simulink model "Test Trajectory"  (R2020a)
settings: Solver=VariableStepAuto  StartTime=0.0  StopTime=10.0  RelTol=1e-3
libraries: simulink x2
settings Model: Creator=ashut  LastModifiedBy=ashut

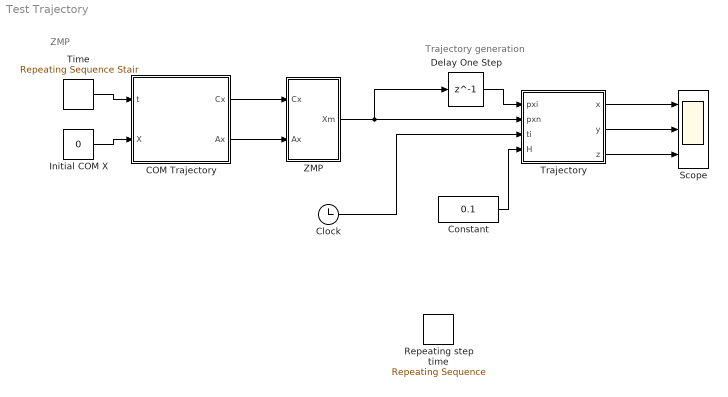
== system Test Trajectory ==
  note: Trajectory generation
  note: ZMP
  COM Trajectory : MATLAB Function  TreatAsAtomicUnit=on
  Clock : Clock
  Constant : Constant  Value=0.1
  Delay One Step : Delay  DelayLength=1
  Initial COM X : Constant  Value=0
  Repeating step time : simulink/Sources/Repeating Sequence  rep_seq_t=[0 0.5]  rep_seq_y=[0 0.5]
  Scope : Scope  NumInputPorts=3
  Time : simulink/Sources/Repeating Sequence Stair  OutValues=[0:1:10].'  tsamp=1  OutMin=[]  OutMax=[]  OutDataTypeStr=double  OutputDataTypeScalingMode=double  OutDataType=fixdt(0,8)  ConRadixGroup=Best Precision: Vector-wise  OutScaling=2^-12
  Trajectory : MATLAB Function  TreatAsAtomicUnit=on
  ZMP : MATLAB Function  TreatAsAtomicUnit=on
  wires:
  COM Trajectory/1(Cx) -> ZMP/1(Cx)
  Constant/1 -> Trajectory/4(H)
  ZMP/1(Xm) -> Delay One Step/1, Trajectory/2(pxn)
  Time/1 -> COM Trajectory/1(t)
  Initial COM X/1 -> COM Trajectory/2(X)
  Delay One Step/1 -> Trajectory/1(pxi)
  COM Trajectory/2(Ax) -> ZMP/2(Ax)
  Trajectory/1(x) -> Scope/1
  Trajectory/2(y) -> Scope/2
  Trajectory/3(z) -> Scope/3
  Clock/1 -> Trajectory/3(ti)

== matlab function Test Trajectory/Trajectory ==
  data: x output; y output; pxi input; z output; pxn input; ti input; H input
function[x,y,z] = Trajectory(pxi,pxn,ti,H)
% pxi is cuttrent x position of endpoint
% pxn is final x position of enpoint
% ti is the real time
% H is the height of the step

% These all are in world frame
step_time = 0.5;
x = pxi + sin((pi/2*step_time)*ti)*abs(pxn-pxi);
y = 0;
z = sin((pi/step_time)*ti)*(H);

== matlab function Test Trajectory/ZMP ==
  data: Cx input; Ax input; Xm output
function Xm  = ZMP(Cx,Ax)

% g and h defined in Parameters.m
% h here is COM height(z-cordinate) from world/path
h = 0.25;
g = 9.8066;
Xm = Cx - (h/g)*(Ax);

== matlab function Test Trajectory/COM Trajectory ==
  data: t input; Cx output; X input; Ax output
function[Cx,Ax] = COM_Trajectory(t,X)
% Here t is sample time
Cx = 0.1*t^2 + X ;
% Vx = 0.2*t;
Ax = 0.2;
